simulink model "p4_signum"  (R2021a)
settings: Solver=VariableStepAuto  StartTime=0.0  StopTime=30  FixedStep=0.00001  RelTol=1e-7
values from neighbouring files (symbols this model uses):
  a = double(a)    [aae666_hw9_p4.m]
  h = 1    [aae666_hw9_p4.m]
undefined symbols (not defined in the file or in its folder): omega
settings Model: Creator=Tomo  LastModifiedBy=Tomo
settings SolverCC: ZeroCrossAlgorithm=Adaptive

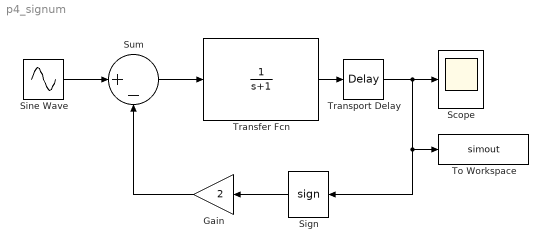
== system p4_signum ==
  Gain : Gain  Gain=2
  Scope : Scope
  Sign : Signum
  Sine Wave : Sin  Amplitude=a  Frequency=omega  SampleTime=0
  Sum : Sum  Inputs=|+-
  To Workspace : ToWorkspace  VariableName=simout  SaveFormat=Structure With Time  SampleTime=-1
  Transfer Fcn : TransferFcn  Denominator=[1 1]
  Transport Delay : TransportDelay  DelayTime=h
  wires:
  Sum/1 -> Transfer Fcn/1
  Sign/1 -> Gain/1
  Gain/1 -> Sum/2
  Sine Wave/1 -> Sum/1
  Transfer Fcn/1 -> Transport Delay/1
  Transport Delay/1 -> To Workspace/1, Sign/1, Scope/1
